simulink model "GasExample_V3"  (R2025b)
settings: Solver=VariableStepAuto  StartTime=0.0  StopTime=1000  RelTol=1e-3
libraries: Bibliothek_FHDO_V1 x14, simulink x6
settings Model: Creator=goessling  LastModifiedBy=goessling

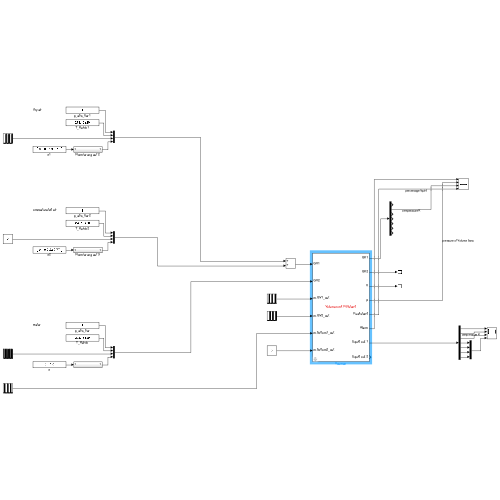
[thumbnail: Simulink's stored preview of the top-level diagram]
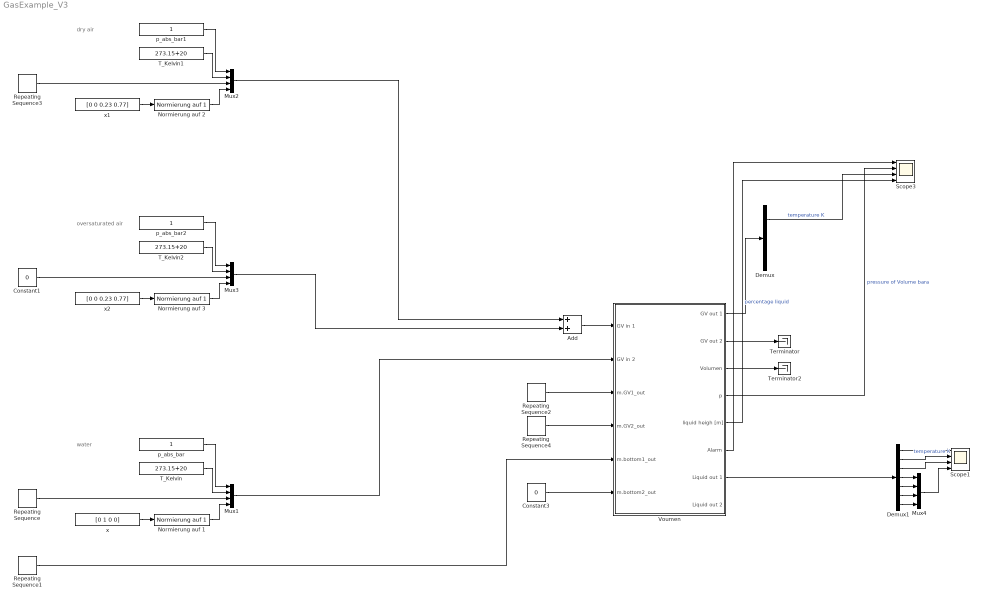
== system GasExample_V3 ==
  note: water
  note: dry air
  note: oversaturated air
  Add : Sum
  Constant1 : Constant  Value=0
  Constant3 : Constant  Value=0
  Demux : Demux  Outputs=7
  Demux1 : Demux  Outputs=7
  Mux{1..4} (4 alike) : Mux
  Normierung auf 1 : Bibliothek_FHDO_V1/Wasser/Normierung auf 1  SystemSampleTime=-1  VariantActivationTime=update diagram  EmptyChoice=off  PassThrough=off  PassThroughVariantControl=(default)  EmptyChoiceVariantControl=(default)  AllowFlexibleInterface=on  Latency=0  AutoFrameSizeCalculation=off
  Normierung auf 2 : Bibliothek_FHDO_V1/Wasser/Normierung auf 1  SystemSampleTime=-1  VariantActivationTime=update diagram  EmptyChoice=off  PassThrough=off  PassThroughVariantControl=(default)  EmptyChoiceVariantControl=(default)  AllowFlexibleInterface=on  Latency=0  AutoFrameSizeCalculation=off
  Normierung auf 3 : Bibliothek_FHDO_V1/Wasser/Normierung auf 1  SystemSampleTime=-1  VariantActivationTime=update diagram  EmptyChoice=off  PassThrough=off  PassThroughVariantControl=(default)  EmptyChoiceVariantControl=(default)  AllowFlexibleInterface=on  Latency=0  AutoFrameSizeCalculation=off
  Repeating Sequence : simulink/Sources/Repeating Sequence  rep_seq_t=[0 100 100.01 500 500.01 600 600.01 1000]  rep_seq_y=[1 1 0 0 1 1 0 0]*282.1778521
  Repeating Sequence1 : simulink/Sources/Repeating Sequence  rep_seq_t=[0 300 300.01 400-1 400.01-1 1000]  rep_seq_y=[0 0 1 1 0 0]*282.1778521
  Repeating Sequence2 : simulink/Sources/Repeating Sequence  rep_seq_t=[0 600 600.01 700 700.01 1000]  rep_seq_y=[0 0 1 1 0 0]*1
  Repeating Sequence3 : simulink/Sources/Repeating Sequence  rep_seq_t=[0 700 700.01 1000]  rep_seq_y=[0 0 1 1]*1
  Repeating Sequence4 : simulink/Sources/Repeating Sequence  rep_seq_t=[0 800 800.01 1000]  rep_seq_y=[0 0 1 1]*1
  Scope1 : Scope  NumInputPorts=4
      settings: ActiveDisplayYMinimum=-1.1885186397454324  ActiveDisplayYMaximum=20.696667757708894
  Scope3 : Scope  NumInputPorts=4
      settings: ActiveDisplayYMinimum=-0.12499999999999997  ActiveDisplayYMaximum=1.125
  T_Kelvin : Constant  Value=273.15+20
  T_Kelvin1 : Constant  Value=273.15+20
  T_Kelvin2 : Constant  Value=273.15+20
  Terminator : Terminator
  Terminator2 : Terminator
  Voumen : Subsystem  mask{A=70685.83471/1000000, h=0.8, p_start=1, T_start=20, x_start=[0 0.014732262 0.229444643 0.755823095], h_start=0}
      mask prompts: A "Area [m^2]"; h "heigh [m]"; p_start "p [bar]"; T_start "T [°C]"; x_start "x"; h_start "liquid level start [m]"
      mask Display:
      | color('red')
      | disp(['Volumen mit Füllstand'])
      | 
      | color('black')
      | port_label('input', 1, 'GV1')
      | port_label('input', 2, 'GV2')
      | port_label('input', 3, 'm.GV1_out')
      | port_label('input', 4, 'm.GV2_out')
      | port_label('input', 5, 'm.bottom1_out')
      | port_label('input', 6, 'm.bottom2_out')
      | 
      | 
      | port_label('output', 1, 'GV1')
      | port_label('output', 2, 'GV2')
      | port_label('output', 3, 'V')
      | port_label('output', 4, 'p')
      | port_label('output', 5, 'Fuellstand')
      | port_label('output', 6, 'Alarm')
      | port_label('output', 7, 'Liquid out 1')
      | port_label('output', 8, 'Liquid out 2')
  p_abs_bar : Constant
  p_abs_bar1 : Constant
  p_abs_bar2 : Constant
  x : Constant  Value=[0 1 0 0]
  x1 : Constant  Value=[0 0 0.23 0.77]
  x2 : Constant  Value=[0 0 0.23 0.77]
  wires:
  Voumen/3(Volumen) -> Terminator2/1
  Voumen/4(p) -> Scope3/2  "pressure of Volume bara"
  Voumen/1(GV out 1) -> Demux/1
  Voumen/2(GV out 2) -> Terminator/1
  Demux/2 -> Scope3/3  "temperature K"
  Voumen/5(liquid heigh [m]) -> Scope3/4  "percentage liquid"
  x/1 -> Normierung auf 1/1
  p_abs_bar/1 -> Mux1/1
  Mux1/1 -> Voumen/2(GV in 2)
  Repeating Sequence/1 -> Mux1/3
  Normierung auf 1/1 -> Mux1/4
  T_Kelvin/1 -> Mux1/2
  T_Kelvin1/1 -> Mux2/2
  Normierung auf 2/1 -> Mux2/4
  Repeating Sequence3/1 -> Mux2/3
  Mux2/1 -> Add/1
  p_abs_bar1/1 -> Mux2/1
  x1/1 -> Normierung auf 2/1
  Mux3/1 -> Add/2
  T_Kelvin2/1 -> Mux3/2
  p_abs_bar2/1 -> Mux3/1
  x2/1 -> Normierung auf 3/1
  Normierung auf 3/1 -> Mux3/4
  Constant1/1 -> Mux3/3
  Add/1 -> Voumen/1(GV in 1)
  Voumen/6(Alarm) -> Scope3/1
  Repeating Sequence1/1 -> Voumen/5(m.bottom1_out)
  Repeating Sequence4/1 -> Voumen/4(m.GV2_out)
  Constant3/1 -> Voumen/6(m.bottom2_out)
  Voumen/7(Liquid out 1) -> Demux1/1
  Demux1/1 -> Scope1/1
  Demux1/2 -> Scope1/2  "temperature K"
  Demux1/3 -> Scope1/3
  Demux1/4 -> Mux4/1
  Demux1/5 -> Mux4/2
  Demux1/6 -> Mux4/3
  Demux1/7 -> Mux4/4
  Mux4/1 -> Scope1/4
  Repeating Sequence2/1 -> Voumen/3(m.GV1_out)

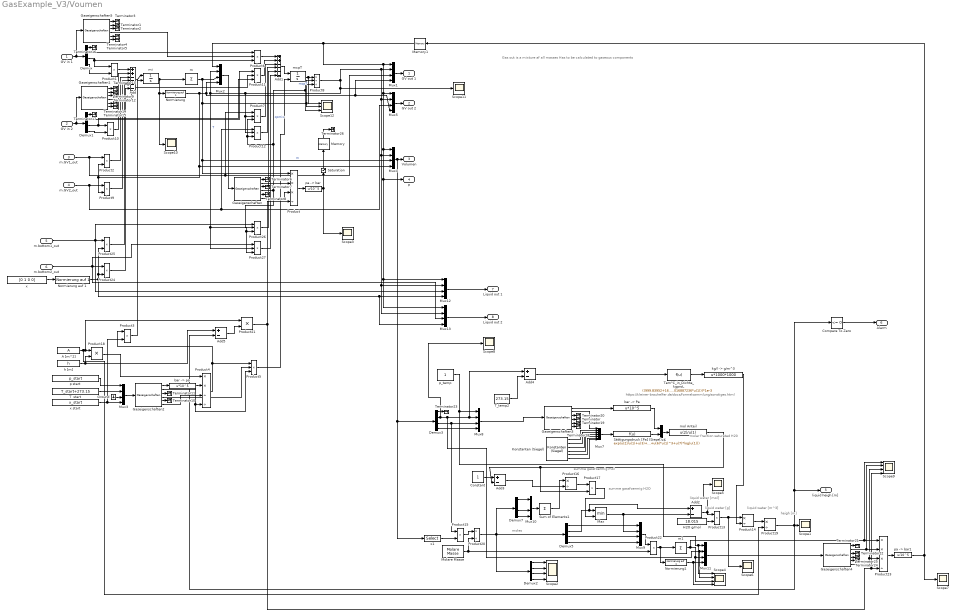
== system GasExample_V3/Voumen ==
  note: Gas out is a mixture af all masses
      | Has to be calculated to gaseous components
  note: https://kleiner-brauhelfer.de/docs/formelsammlung/sonstiges.html
  note: molar fraction saturated H20
  note: moles
  note: liquid water [mol]
  note: summe gassfoermig mol
  note: summe gassfoermig H2O
  note: liquid water [m^3]
  note: heigh [m]
  note: liquid water [g]
  GV in 1 : Inport
  GV in 2 : Inport  Port=2
  m.GV1_out : Inport  Port=3
  m.GV2_out : Inport  Port=4
  m.bottom1_out : Inport  Port=5
  m.bottom2_out : Inport  Port=6
  A [m^2] : Constant  Value=A
  Add : Sum  Inputs=++----
  Add1 : Sum  Inputs=++----  SampleTime=.01
  Add{2..5} (4 alike) : Sum  Inputs=+-
  Compare To Zero : simulink/Logic and Bit Operations/Compare To Zero  relop=<=  OutDataTypeStr=boolean
  Constant : Constant
  Demux : Demux  Outputs=[1 1 1 4]
  Demux1 : Demux  Outputs=[1 1 1 4]
  Demux2 : Demux  Outputs=[1 1 1 1]
  Demux3 : Demux  Outputs=[1 1 1 4]
  Demux5 : Demux  Outputs=[1 1 1 1]
  Demux7 : Demux  Outputs=[1 1 1 1]
  Gaseigenschaften{,1..5} (6 alike) : Bibliothek_FHDO_V1/Gaseigenschaften  SystemSampleTime=-1  VariantActivationTime=update diagram  EmptyChoice=off  PassThrough=off  PassThroughVariantControl=(default)  EmptyChoiceVariantControl=(default)  AllowFlexibleInterface=on  Latency=0  AutoFrameSizeCalculation=off
  Ground : Ground
  H2O g/mol : Constant  Value=18.015
  Konstanten (Siegel) : Bibliothek_FHDO_V1/Befeuchter//Abscheider/Konstanten (Siegel)  SystemSampleTime=-1  VariantActivationTime=update diagram  EmptyChoice=off  PassThrough=off  PassThroughVariantControl=(default)  EmptyChoiceVariantControl=(default)  AllowFlexibleInterface=on  Latency=0  AutoFrameSizeCalculation=off
  Max : MinMax  Inputs=2
  Memory : Memory  InitialCondition=p_start
  Memory1 : Memory  InitialCondition=p_start
  Molare Masse : Bibliothek_FHDO_V1/Gaseigenschaften/Molare Masse  SystemSampleTime=-1  VariantActivationTime=update diagram  EmptyChoice=off  PassThrough=off  PassThroughVariantControl=(default)  EmptyChoiceVariantControl=(default)  AllowFlexibleInterface=on  Latency=0  AutoFrameSizeCalculation=off
  Mux{1..5,8..13} (11 alike) : Mux
  Mux6 : Mux  Inputs=2
  Mux7 : Mux  Inputs=7
  Normierung : Bibliothek_FHDO_V1/Sauerstoff/Normierung auf 1  SystemSampleTime=-1  VariantActivationTime=update diagram  EmptyChoice=off  PassThrough=off  PassThroughVariantControl=(default)  EmptyChoiceVariantControl=(default)  AllowFlexibleInterface=on  Latency=0  AutoFrameSizeCalculation=off
  Normierung auf 1 : Bibliothek_FHDO_V1/Wasser/Normierung auf 1  SystemSampleTime=-1  VariantActivationTime=update diagram  EmptyChoice=off  PassThrough=off  PassThroughVariantControl=(default)  EmptyChoiceVariantControl=(default)  AllowFlexibleInterface=on  Latency=0  AutoFrameSizeCalculation=off
  Normierung1 : Bibliothek_FHDO_V1/Sauerstoff/Normierung auf 1  SystemSampleTime=-1  VariantActivationTime=update diagram  EmptyChoice=off  PassThrough=off  PassThroughVariantControl=(default)  EmptyChoiceVariantControl=(default)  AllowFlexibleInterface=on  Latency=0  AutoFrameSizeCalculation=off
  Product : Product  Inputs=***/  RndMeth=Zero
  Product{1..3,9..10,13,15,17,24..25} (10 alike) : Product  RndMeth=Zero
  Product{5..7,11..12,26..27} (7 alike) : Product  Inputs=3  RndMeth=Zero
  Product{14,16,19..20} (4 alike) : Product  Inputs=*/  RndMeth=Zero
  Product18 : Product
  Product21 : Product
  Product22 : Product  Inputs=**  RndMeth=Zero
  Product23 : Product  Inputs=***/  RndMeth=Zero
  Product4 : Product  Inputs=**//  RndMeth=Zero
  Product8 : Product  Inputs=*//  RndMeth=Zero
  Saturation : Saturate  UpperLimit=inf  LowerLimit=1
  Scope{1,3,5..8,10..11} (8 alike) : Scope
      Scope1 settings: ActiveDisplayYMinimum=0.1217  ActiveDisplayYMaximum=0.53228
      Scope10 settings: ActiveDisplayYMinimum=-3527.53472  ActiveDisplayYMaximum=31747.81251  DataLoggingVariableName=ScopeData2
      Scope11 settings: ActiveDisplayYMinimum=289.4277  ActiveDisplayYMaximum=326.65069  DataLoggingVariableName=ScopeData3
      Scope3 settings: ActiveDisplayYMinimum=-6.693421776112315E+14  ActiveDisplayYMaximum=5.1024681544999231E+14  DataLoggingVariableName=ScopeData3
      Scope5 settings: ActiveDisplayYMinimum=-624.70213  ActiveDisplayYMaximum=5622.3192  DataLoggingVariableName=ScopeData5
      Scope6 settings: ActiveDisplayYMinimum=-11254.00894  ActiveDisplayYMaximum=101286.08044  DataLoggingVariableName=ScopeData2
      Scope7 settings: ActiveDisplayYMinimum=-1.5251632441880252E+11  ActiveDisplayYMaximum=5.46273191750929E+10  DataLoggingVariableName=ScopeData5
      Scope8 settings: ActiveDisplayYMinimum=263.30209  ActiveDisplayYMaximum=361.78123  DataLoggingVariableName=ScopeData6
  Scope12 : Scope  NumInputPorts=3
      settings: ActiveDisplayYMinimum=-1.92104645928E+6  ActiveDisplayYMaximum=1.750985915796E+7  DataLoggingVariableName=ScopeData4
  Scope2 : Scope  NumInputPorts=4
      settings: ActiveDisplayYMinimum=-1  ActiveDisplayYMaximum=1
  Scope4 : Scope  NumInputPorts=4
      settings: ActiveDisplayYMinimum=0.9  ActiveDisplayYMaximum=1.1  DataLoggingVariableName=ScopeData4
  Scope9 : Scope  NumInputPorts=4
      settings: ActiveDisplayYMinimum=73.42301  ActiveDisplayYMaximum=73.4232  DataLoggingVariableName=ScopeData7
  Sum of Elements1 : Sum  Inputs=+
  Sättigungsdruck [Pa] (Siegel) : Fcn  Expr=exp(u(2)/u(1)+u(3)+u(4)*u(1)+u(5)*u(1)^2+u(6)*u(1)^3+u(7)*log(u(1)))
  T  start : Constant  Value=T_start+273.15
  T_temp2 : Constant  Value=273.15
  Tem°C_in_Dichte_kgproL : Fcn  Expr=((999.83952+16.952577*u(1)-0.0079905127*u(1)^2-0.000046241757*u(1)^3+0.00000010584601*u(1)^4-0.00000000028103006*u(1)^5)/(1+0.016887236*u(1)))*1e-3
  Terminator{,1..26} (27 alike) : Terminator
  "bar -> Pa" : Fcn  Expr=u*10^5
  "bar -> pa" : Fcn  Expr=u*10^5
  h [m] : Constant  Value=h
  "kg/l -> g/m^3" : Fcn  Expr=u*1000*1000
  m : Sum  Inputs=+
  m1 : Sum  Inputs=+
  mcpT : Integrator  InitialConditionSource=external  InitialCondition=[0 0 0 0 0 0 .21 .79]*1293
  mi : Integrator  InitialConditionSource=external  InitialCondition=[0 0 0 0 0 0 .21 .79]*1293
  mol Anteil : Fcn  Expr=u(2)/u(1)
  p start : Constant  Value=p_start
  p_temp : Constant
  "pa -> bar" : Fcn  Expr=u/10^5
  "pa -> bar1" : Fcn  Expr=u/10^5
  x : Constant  Value=[0 1 0 0]
  x start : Constant  Value=x_start
  x1 : Selector  InputPortWidth=7  IndexOptions=Index vector (dialog)  Indices=[4 5 6 7]  OutputSizes=1
  GV out 1 : Outport
  GV out 2 : Outport  Port=2
  Volumen : Outport  Port=3
  p : Outport  Port=4
  liquid heigh [m] : Outport  Port=5
  Alarm : Outport  Port=6
  Liquid out 1 : Outport  Port=7
  Liquid out 2 : Outport  Port=8
  wires:
  GV in 1/1 -> Gaseigenschaften5/1, Demux/1
  Demux/3 -> Product1/1, Product6/3
  Demux/2 -> Product6/1
  Demux/4 -> Product1/2
  Gaseigenschaften/1 -> Terminator6/1
  Gaseigenschaften/4 -> Product27/3, Product26/3, Product8/3, Scope12/3, Product7/3, Product12/3  "cpmix"
  Product1/1 -> Add/1
  m.GV1_out/1 -> Product2/1, Product7/1, Mux1/3
  Normierung/1 -> Mux2/4, Mux1/4, Mux5/4, Mux4/4, Product2/2, Product9/2
  Product2/1 -> Add/3
  Add/1 -> mi/1
  m/1 -> Mux2/3, Product8/2, Scope12/2, Product/1, Mux4/3  "m"
  Gaseigenschaften5/1 -> Terminator3/1
  Gaseigenschaften5/4 -> Product6/2
  Gaseigenschaften/6 -> Product/3
  Gaseigenschaften/2 -> Product/2
  A [m^2]/1 -> Product19/2, Product21/1, Product18/1
  Product/1 -> "pa -> bar"/1
  Mux1/1 -> GV out 1/1
  Gaseigenschaften5/2 -> Terminator1/1
  Gaseigenschaften5/3 -> Terminator2/1
  Gaseigenschaften5/5 -> Terminator4/1
  Gaseigenschaften5/6 -> Terminator5/1
  Gaseigenschaften/3 -> Terminator7/1
  Gaseigenschaften/5 -> Terminator8/1
  x start/1 -> Mux3/4, Product3/2
  Ground/1 -> Mux3/3
  p start/1 -> Mux3/1
  T  start/1 -> Mux3/2
  Mux3/1 -> Gaseigenschaften2/1
  Gaseigenschaften2/1 -> "bar -> pa"/1
  "bar -> pa"/1 -> Product4/2
  Gaseigenschaften2/6 -> Product4/3
  Gaseigenschaften2/2 -> Product4/4, Product5/3
  Gaseigenschaften2/3 -> Terminator11/1
  Gaseigenschaften2/4 -> Product5/2
  Gaseigenschaften2/5 -> Terminator10/1
  Product4/1 -> Product5/1, Product3/1
  Product3/1 -> mi/2
  Product5/1 -> mcpT/2
  Product6/1 -> Add1/1
  Add1/1 -> mcpT/1
  mcpT/1 -> Scope12/1, Product8/1  "mcpT"
  Product8/1 -> Product27/2, Product26/2, Mux2/2, Product7/2, Product12/2, Scope11/1, Mux1/2, Mux13/2, Mux12/2, Mux4/2, Mux5/2  "T"
  Product7/1 -> Add1/3
  m.GV2_out/1 -> Product9/1, Mux5/3, Product12/1
  Product9/1 -> Add/4
  Mux5/1 -> GV out 2/1
  GV in 2/1 -> Gaseigenschaften1/1, Demux1/1
  Gaseigenschaften1/1 -> Terminator13/1
  Gaseigenschaften1/2 -> Terminator9/1
  Gaseigenschaften1/3 -> Terminator12/1
  Gaseigenschaften1/5 -> Terminator14/1
  Gaseigenschaften1/6 -> Terminator15/1
  Demux/1 -> Terminator16/1
  Demux1/1 -> Terminator17/1
  Demux1/3 -> Product10/1, Product11/3
  Demux1/4 -> Product10/2
  Product10/1 -> Add/2
  Product11/1 -> Add1/2
  Product12/1 -> Add1/4
  Gaseigenschaften1/4 -> Product11/2
  Demux1/2 -> Product11/1
  Saturation/1 -> Memory/1
  Mux6/1 -> mol Anteil/1
  Sättigungsdruck [Pa] (Siegel)/1 -> Mux6/2
  Gaseigenschaften3/5 -> Terminator19/1
  Gaseigenschaften3/6 -> Terminator18/1
  Gaseigenschaften3/3 -> Terminator20/1
  Mux4/1 -> x1/1, Demux3/1, Volumen/1
  Gaseigenschaften3/1 -> "bar -> Pa"/1
  mol Anteil/1 -> Product17/2, Add3/2
  Konstanten (Siegel)/1 -> Mux7/2
  Gaseigenschaften3/2 -> Mux7/1
  Konstanten (Siegel)/6 -> Mux7/7
  "bar -> Pa"/1 -> Mux6/1
  Konstanten (Siegel)/3 -> Mux7/4
  Gaseigenschaften3/4 -> Terminator/1
  Mux7/1 -> Sättigungsdruck [Pa] (Siegel)/1
  Konstanten (Siegel)/4 -> Mux7/5
  Konstanten (Siegel)/5 -> Mux7/6
  Konstanten (Siegel)/2 -> Mux7/3
  p_temp/1 -> Scope4/1, Mux11/1, Mux8/1
  Demux3/3 -> Mux8/3, Product15/1
  Demux3/4 -> Mux8/4
  Demux3/1 -> Terminator23/1
  Mux8/1 -> Gaseigenschaften3/1
  Demux2/1 -> Scope2/1
  Demux2/2 -> Scope2/2
  Demux2/3 -> Scope2/3
  Demux2/4 -> Scope2/4
  mi/1 -> Scope10/1, Normierung/1, m/1
  x1/1 -> Product15/2
  Demux5/2 -> Add2/1, Max/1
  Demux5/1 -> Mux9/1
  Demux5/3 -> Mux9/3
  Demux5/4 -> Mux9/4
  Max/1 -> Mux9/2, Add2/2
  Add2/1 -> Product13/1, Scope5/1
  Constant/1 -> Add3/1
  Demux7/1 -> Mux10/1
  Demux7/3 -> Mux10/3
  Demux7/4 -> Mux10/4
  Mux10/1 -> Sum of Elements1/1
  Sum of Elements1/1 -> Product16/1
  Add3/1 -> Product16/2
  Product16/1 -> Product17/1
  Product17/1 -> Max/2
  h [m]/1 -> Add5/1, Product18/2
  H2O g/mol/1 -> Product13/2
  Tem°C_in_Dichte_kgproL/1 -> "kg/l -> g/m^3"/1
  Product13/1 -> Scope6/1, Product14/1
  "kg/l -> g/m^3"/1 -> Product14/2
  Product14/1 -> Product19/1
  Product19/1 -> Compare To Zero/1, liquid heigh [m]/1, Add5/2, Scope1/1
  Product15/1 -> Product20/1
  Product20/1 -> Demux2/1, Demux5/1, Demux7/1
  Molare Masse/1 -> Product22/2, Product20/2
  T_temp2/1 -> Add4/2
  Add4/1 -> Tem°C_in_Dichte_kgproL/1
  Add5/1 -> Product21/2
  Product21/1 -> Product23/4, Scope9/4, Product/4
  Product18/1 -> Product4/1
  "pa -> bar"/1 -> Saturation/1, Scope3/1
  Mux9/1 -> Product22/1
  Product22/1 -> Normierung1/1, m1/1
  m1/1 -> Scope9/1, Product23/1, Scope4/3, Mux11/3
  Normierung1/1 -> Scope4/4, Mux11/4
  Mux2/1 -> Gaseigenschaften/1
  Mux11/1 -> Gaseigenschaften4/1
  Gaseigenschaften4/1 -> Terminator21/1
  Gaseigenschaften4/3 -> Terminator22/1
  Gaseigenschaften4/5 -> Terminator24/1
  Gaseigenschaften4/2 -> Scope9/2, Product23/2
  Gaseigenschaften4/4 -> Terminator25/1
  Gaseigenschaften4/6 -> Product23/3, Scope9/3
  Product23/1 -> "pa -> bar1"/1
  Demux3/2 -> Scope4/2, Mux11/2, Add4/1, Mux8/2, Scope8/1
  "pa -> bar1"/1 -> Memory1/1, Scope7/1
  Memory1/1 -> Mux1/1, Mux5/1, Mux4/1, Mux13/1, Mux12/1, p/1, Mux2/1
  Memory/1 -> Terminator26/1
  x/1 -> Normierung auf 1/1
  Normierung auf 1/1 -> Mux13/4, Mux12/4, Product25/2, Product24/2
  m.bottom2_out/1 -> Product27/1, Mux13/3, Product24/1
  m.bottom1_out/1 -> Product26/1, Mux12/3, Product25/1
  Product25/1 -> Add/5
  Product24/1 -> Add/6
  Mux12/1 -> Liquid out 1/1
  Mux13/1 -> Liquid out 2/1
  Compare To Zero/1 -> Alarm/1
  Product26/1 -> Add1/5
  Product27/1 -> Add1/6
